simulink model "PvsPIvsPID"  (R2023a)
settings: Solver=VariableStepAuto  StartTime=0.0  StopTime=2800  RelTol=1e-3
values from neighbouring files (symbols this model uses):
  F2 = 6.32    [ConstantesCPQ23m.m]    (also in lugardasRaizes.m)
  K = J/(Tau*wn2)    [ConstantesCPQ23m.m]    (also in lugardasRaizes.m)
  qsi = (P/Tau)/(2*wn)    [ConstantesCPQ23m.m]    (also in lugardasRaizes.m)
  wn = sqrt(1/Tau)    [ConstantesCPQ23m.m]    (also in lugardasRaizes.m)
  wn2 = (1/Tau)    [ConstantesCPQ23m.m]    (also in lugardasRaizes.m)
settings Model: Creator=Estudo  LastModifiedBy=Estudo

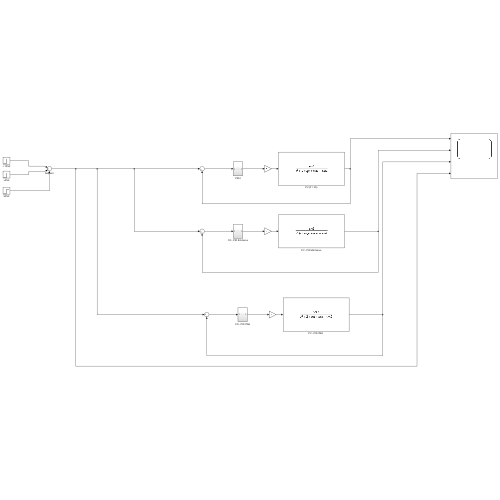
[thumbnail: Simulink's stored preview of the top-level diagram]
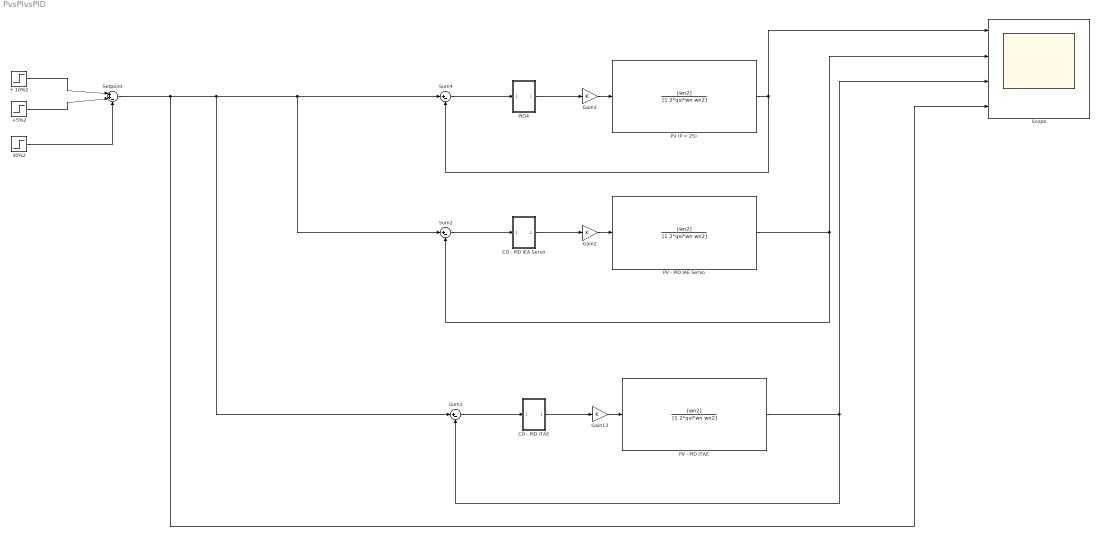
== system PvsPIvsPID ==
  + 10%2 : Step  After=F2 + F2*0.1  SampleTime=0
  +5%2 : Step  Time=1200  After=F2*0.05  SampleTime=0
  30%2 : Step  Time=2000  After=F2*0.3  SampleTime=0
  CO - PID IEA Servo : Subsystem
  CO - PID ITAE : Subsystem
  Gain13 : Gain  Gain=K
  Gain2 : Gain  Gain=K
  Gain3 : Gain  Gain=K
  PID4 : Subsystem
  PV (P = 25) : TransferFcn  Numerator=[wn2]  Denominator=[1 2*qsi*wn wn2]
  PV - PID IAE Servo : TransferFcn  Numerator=[wn2]  Denominator=[1 2*qsi*wn wn2]
  "PV - PID ITAE " : TransferFcn  Numerator=[wn2]  Denominator=[1 2*qsi*wn wn2]
  Scope : Scope  NumInputPorts=4
  Setpoint : Sum  Inputs=|++-
  Sum2 : Sum  Inputs=|+-
  Sum3 : Sum  Inputs=|+-
  Sum4 : Sum  Inputs=|+-
  wires:
  30%2/1 -> Setpoint/3
  +5%2/1 -> Setpoint/2
  + 10%2/1 -> Setpoint/1
  Gain3/1 -> PV (P = 25)/1
  PID4/1(Out1) -> Gain3/1
  Sum4/1 -> PID4/1(In1)
  PV (P = 25)/1 -> Sum4/2, Scope/1
  CO - PID IEA Servo/1(Out1) -> Gain2/1
  Sum2/1 -> CO - PID IEA Servo/1(In1)
  PV - PID IAE Servo/1 -> Scope/2, Sum2/2
  Gain2/1 -> PV - PID IAE Servo/1
  "PV - PID ITAE "/1 -> Scope/3, Sum3/2
  Gain13/1 -> "PV - PID ITAE "/1
  Sum3/1 -> CO - PID ITAE/1(In1)
  CO - PID ITAE/1(Out1) -> Gain13/1
  Setpoint/1 -> Scope/4, Sum3/1, Sum2/1, Sum4/1

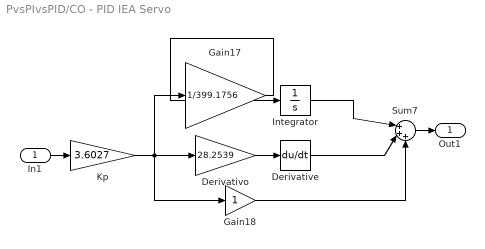
== system PvsPIvsPID/CO - PID IEA Servo ==
  In1 : Inport
  Derivative : Derivative
  Derivativo : Gain  Gain=28.2539
  Gain17 : Gain  Gain=1/399.1756
  Gain18 : Gain
  Integrator : Integrator
  Kp : Gain  Gain=3.6027
  Sum7 : Sum  Inputs=|+++
  Out1 : Outport
  wires:
  Gain18/1 -> Sum7/3
  Integrator/1 -> Sum7/1
  Kp/1 -> Gain17/1, Gain18/1, Derivativo/1
  Derivativo/1 -> Derivative/1
  In1/1 -> Kp/1
  Gain17/1 -> Integrator/1
  Derivative/1 -> Sum7/2
  Sum7/1 -> Out1/1

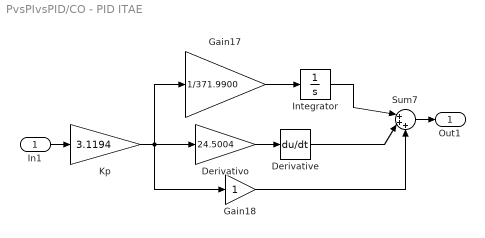
== system PvsPIvsPID/CO - PID ITAE ==
  In1 : Inport
  Derivative : Derivative
  Derivativo : Gain  Gain=24.5004
  Gain17 : Gain  Gain=1/371.9900
  Gain18 : Gain
  Integrator : Integrator
  Kp : Gain  Gain=3.1194
  Sum7 : Sum  Inputs=|+++
  Out1 : Outport
  wires:
  Gain18/1 -> Sum7/3
  Integrator/1 -> Sum7/1
  Kp/1 -> Gain18/1, Gain17/1, Derivativo/1
  Derivativo/1 -> Derivative/1
  In1/1 -> Kp/1
  Gain17/1 -> Integrator/1
  Derivative/1 -> Sum7/2
  Sum7/1 -> Out1/1

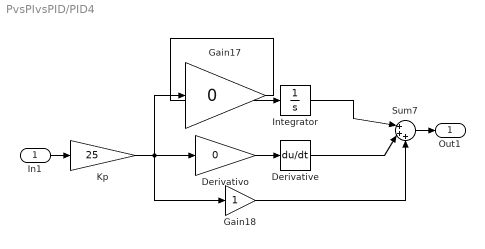
== system PvsPIvsPID/PID4 ==
  In1 : Inport
  Derivative : Derivative
  Derivativo : Gain  Gain=0
  Gain17 : Gain  Gain=0
  Gain18 : Gain
  Integrator : Integrator
  Kp : Gain  Gain=25
  Sum7 : Sum  Inputs=|+++
  Out1 : Outport
  wires:
  Gain18/1 -> Sum7/3
  Integrator/1 -> Sum7/1
  Kp/1 -> Gain17/1, Gain18/1, Derivativo/1
  Derivativo/1 -> Derivative/1
  In1/1 -> Kp/1
  Gain17/1 -> Integrator/1
  Derivative/1 -> Sum7/2
  Sum7/1 -> Out1/1
